simulink model "modelo_BDA"  (R2021b)
settings: Solver=ode3  StartTime=0.0  StopTime=10.0  FixedStep=1e-6  RelTol=1e-3
(part 4 of 4)

== matlab function modelo_BDA/U ==
  data: q input; U output
function U = U(q)
%#codegen

q1 = q(1);
q2 = q(2);
q3 = q(3);
q4 = q(4);
q5 = q(5);
q6 = q(6);
%    This function was generated by the Symbolic Math Toolbox version 9.0.
%    01-Dec-2021 19:55:58

t2 = cos(q1);
t3 = cos(q2);
t4 = cos(q4);
t5 = cos(q5);
t6 = cos(q6);
t7 = sin(q1);
t8 = sin(q2);
t9 = sin(q4);
t10 = sin(q5);
t11 = sin(q6);
t12 = q1+q2;
t18 = 9.007199254740992e+15;
t13 = cos(t12);
t14 = sin(t12);
t20 = (q3.*t18)./9.007199254740992e+15;
t23 = q3.*t18.*1.110223024625157e-16i;
t15 = t14.*4.602992943936994e+15;
t16 = t13.*7.742227997977903e+15;
t21 = cos(t20);
t22 = sin(t20);
t24 = exp(t23);
t25 = -t23;
t17 = -t15;
t26 = 1.0./t24;
t27 = t22.*1i;
t28 = t24-1.0;
t33 = t21.*7.38843356682345e-1;
t34 = t21.*2.61156643317655e-1;
t36 = t4.*t18.*t22.*(t15-t16).*(-1.232595164407831e-32);
t37 = t9.*t18.*t22.*(t15-t16).*(-1.232595164407831e-32);
t38 = (t4.*t18.*t22.*(t15-t16))./8.112963841460668e+31;
t19 = t16+t17;
t29 = -t27;
t30 = t28.^2;
t32 = t21+t27-1.0;
t39 = t33+2.61156643317655e-1;
t40 = t34+7.38843356682345e-1;
t31 = t21+t29;
t35 = t32.^2;
t41 = t13.*t39;
t42 = t14.*t40;
t43 = t13.*t31.*t35.*2.196325630278387e-1;
t44 = t14.*t31.*t35.*2.196325630278387e-1;
t45 = -t43;
t46 = -t44;
t47 = t41+t46;
t48 = t42+t45;
t49 = t4.*t48;
t50 = t5.*t47;
t51 = t9.*t48;
t52 = t37+t49;
t53 = t38+t51;
t54 = t10.*t53;
t55 = -t54;
t56 = t50+t55;
et1 = t2.*9.734313510982566e+7-t7.*2.717189225818344e+7;
et2 = t13.*3.161091753815448e+6+t14.*4.486343276457132e+6;
et3 = t41.*1.120052718265734e+7+t42.*9.403213850994834e+5;
et4 = t49.*1.663770937481834e+6+t50.*1.034557445559048e+6;
et5 = t51.*(-1.835160358667313e+3)-t54.*1.034557445559048e+6;
et6 = t2.*t3.*1.83714624816208e+7;
et7 = t2.*t8.*2.794679323535407e+7;
et8 = t3.*t7.*2.794679323535407e+7;
et9 = t7.*t8.*(-1.83714624816208e+7);
et10 = t10.*t47.*1.330750753053523e+6+t5.*t53.*1.330750753053523e+6;
et11 = t6.*t52.*7.125500496317142e+5+t6.*t56.*1.310984838335871e+6;
et12 = t11.*t52.*(-1.310984838335871e+6)+t11.*t56.*7.125500496317142e+5;
et13 = t2.*t3.*t21.*7.745725473871877e+6;
et14 = t2.*t8.*t21.*(-4.605072301050445e+6);
et15 = t3.*t7.*t21.*(-4.605072301050445e+6);
et16 = t7.*t8.*t21.*(-7.745725473871877e+6);
et17 = t13.*t26.*t30.*(-2.065251958792868e+5);
et18 = t14.*t26.*t30.*(-1.021066241114224e+6);
et19 = t14.*t31.*t35.*(-1.438934251275785e+6);
et20 = t2.*t3.*t18.*t22.*1.61551131708884e-17;
et21 = t2.*t8.*t18.*t22.*(-9.604712229286526e-18);
et22 = t3.*t7.*t18.*t22.*(-9.604712229286526e-18);
et23 = t7.*t8.*t18.*t22.*(-1.61551131708884e-17);
et24 = t4.*t18.*t22.*(t15-t16).*(-2.262009784006271e-29);
et25 = t9.*t18.*t22.*(t15-t16).*(-2.050756012222393e-26);
U = et1+et2+et3+et4+et5+et6+et7+et8+et9+et10+et11+et12+et13+et14+et15+et16+et17+et18+et19+et20+et21+et22+et23+et24+et25;
